simulink model "sampleModel89"  (R2021b)
settings: Solver=VariableStepAuto  StartTime=0.0  StopTime=10.0  RelTol=1e-3
undefined symbols (not defined in the file or in its folder): magnitude
libraries: simulink x7
settings Model: Creator=user  LastModifiedBy=user

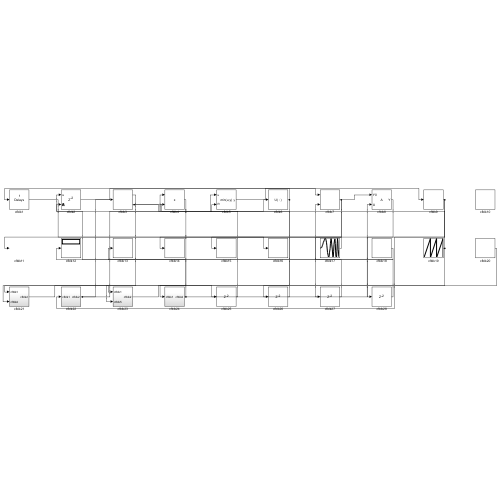
[thumbnail: Simulink's stored preview of the top-level diagram]
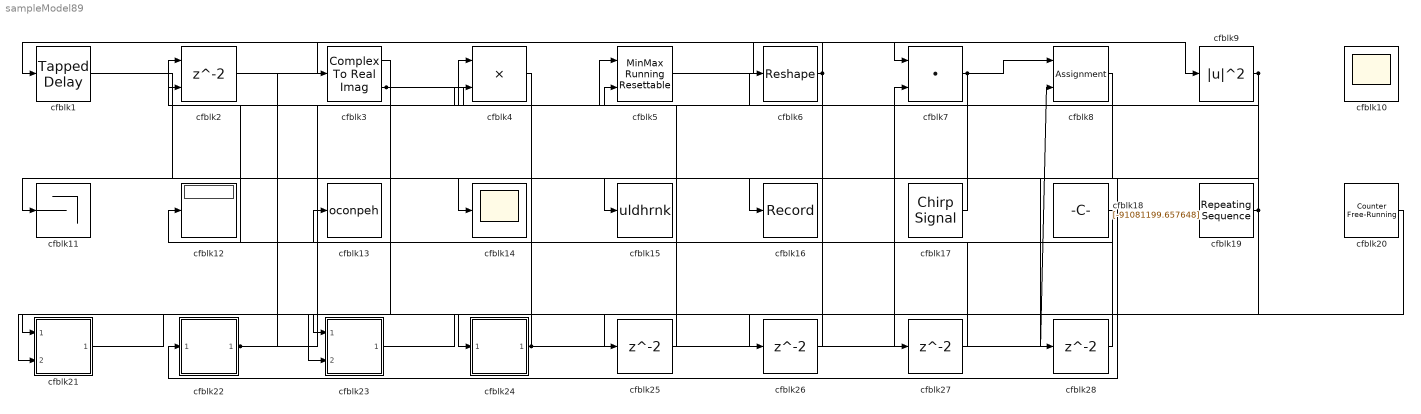
== system sampleModel89 ==
  cfblk1 : simulink/Discrete/Tapped Delay  vinit=0.0  samptime=-1  NumDelays=1  DelayOrder=Oldest  includeCurrent=off
  cfblk10 : Scope
      settings: Floating=on
  cfblk11 : Terminator
  cfblk12 : Display
  cfblk13 : ToWorkspace  VariableName=oconpeh  SaveFormat=Timeseries  SampleTime=-1
  cfblk14 : Scope
  cfblk15 : ToWorkspace  VariableName=uldhrnk  SaveFormat=Timeseries  SampleTime=-1
  cfblk16 : Record  FileSettingsInternal="{\"entries\":[{\"content\":{\"excelSettings\":{\"content\":{},\"type\":\"Streamout.ExcelSettings\"}},\"type\":\"Streamout.FileSettingStorage\",\"uuid\":\"fac87c34-e0b7-4349-b6f4-70da045e78e1\"}],\"packageUris\":[\"http://schema.mathworks.com/mf0/streamout_blocks/R2020a\"],\"version\":\"1.0\"}"  SignalsInternal="{\"entries\":[{\"content\":{\"signals\":[{\"content\":{\"blockPath\":[\"sampleModel89/cfblk16\"],\"channel\":[],\"dimensions\":[1],\"domain\":\"sampleModel89/cfblk16\",\"lineColor\":\"#a2142f\",\"plots\":[1],\"port\":1,\"sid\":[\"\"],\"signalID\":3255,\"signalName\":\"cfblk1\"},\"type\":\"RecordBlkView.Signal\",\"uuid\":\"2643ba45-9ab1-445a-bdcd-ba3203e13d56\"}]},\"type\":\"RecordBlkView.InputSignals\",\"uuid\":\"61955a5d-bbc7-4503-a666-7dac71005f09\"}],\"packageUris\":[\"http://schema.mathworks.com/mf0/streamout_blocks/R2020a\"],\"version\":\"1.0\"}"  VisualizationBindings="{\"sparklinesplugin\":{\"info\":[{\"bindingParametersList\":[],\"subplotID\":1}]}}"
  cfblk17 : simulink/Sources/Chirp Signal  f1=[-255475607.936733]  T=[740321862.264641]  f2=[288984347.187765]
  cfblk18 : Constant  Value=[-91081199.657648]  SampleTime=1
  cfblk19 : simulink/Sources/Repeating Sequence  rep_seq_t=[0 2]  rep_seq_y=[-500814716.924603, 310036400.015080]
  cfblk2 : Delay  ShowEnablePort=on  SampleTime=1
      settings: InputPortMap=u0,e6
  cfblk20 : simulink/Sources/Counter Free-Running  NumBits=[30.000000]  tsamp=-1
  cfblk21 : Subsystem
  cfblk22 : Subsystem
  cfblk23 : Subsystem
  cfblk24 : Subsystem
  cfblk{25..28} (4 alike) : Delay  SampleTime=1
  cfblk3 : ComplexToRealImag
  cfblk4 : Product  Inputs=**
  cfblk5 : simulink/Math Operations/MinMax Running Resettable  Function=min  vinit=0.0
  cfblk6 : Reshape
  cfblk7 : DotProduct  InputSameDT=on  OutDataTypeStr=Inherit: Inherit via internal rule
  cfblk8 : Assignment  DiagnosticForDimensions=Warning  IndexOptions=Index vector (dialog)  Indices=1  OutputSizes=1
  cfblk9 : Math  Operator=magnitude^2  SaturateOnIntegerOverflow=on
  wires:
  cfblk2/1 -> cfblk9/1
  cfblk17/1 -> cfblk11/1
  cfblk18/1 -> cfblk12/1
  cfblk7/1 -> cfblk8/1, cfblk14/1, cfblk26/1
  cfblk5/1 -> cfblk7/1
  cfblk6/1 -> cfblk1/1, cfblk15/1
  cfblk22/1(cfblk2) -> cfblk4/1, cfblk3/1
  cfblk4/1 -> cfblk21/1(cfblk1)
  cfblk24/1(cfblk2) -> cfblk13/1, cfblk8/2
  cfblk9/1 -> cfblk22/1(cfblk1), cfblk28/1
  cfblk1/1 -> cfblk16/1
  cfblk21/1(cfblk2) -> cfblk23/1(cfblk1)
  cfblk19/1 -> cfblk2/1, cfblk24/1(cfblk1)
  cfblk3/1 -> cfblk21/2(cfblk4)
  cfblk3/2 -> cfblk5/2, cfblk6/1
  cfblk20/1 -> cfblk23/2(cfblk5)
  cfblk23/1(cfblk2) -> cfblk25/1
  cfblk25/1 -> cfblk4/2
  cfblk26/1 -> cfblk5/1
  cfblk8/1 -> cfblk27/1
  cfblk27/1 -> cfblk7/2
  cfblk28/1 -> cfblk2/2

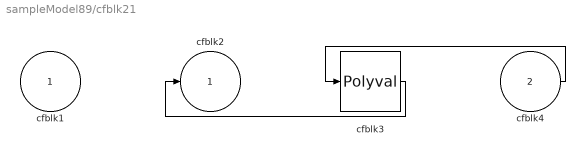
== system sampleModel89/cfblk21 ==
  cfblk1 : Inport
  cfblk4 : Inport  Port=2
  cfblk3 : Polyval  Coefs=[ +2.081618890e-019, -1.441693666e-014, +4.719686976e-010, -8.536869453e-006, +1.621573104e-001, -8.087801117e+001 ]
  cfblk2 : Outport
  wires:
  cfblk4/1 -> cfblk3/1
  cfblk3/1 -> cfblk2/1

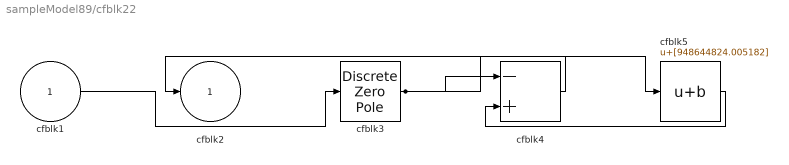
== system sampleModel89/cfblk22 ==
  cfblk1 : Inport
  cfblk3 : DiscreteZeroPole  Poles=[0 0.5]  Gain=1
  cfblk4 : Sum  Inputs=-+
  cfblk5 : Bias  Bias=[948644824.005182]
  cfblk2 : Outport
  wires:
  cfblk4/1 -> cfblk2/1
  cfblk1/1 -> cfblk3/1
  cfblk3/1 -> cfblk4/1, cfblk5/1
  cfblk5/1 -> cfblk4/2

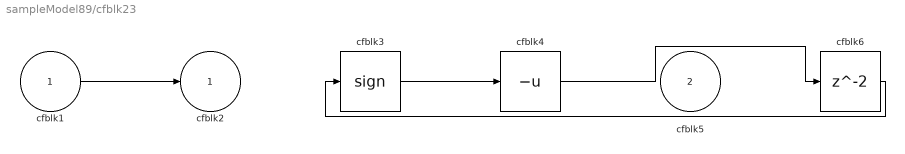
== system sampleModel89/cfblk23 ==
  cfblk1 : Inport
  cfblk5 : Inport  Port=2
  cfblk3 : Signum
  cfblk4 : UnaryMinus
  cfblk6 : Delay  SampleTime=1
  cfblk2 : Outport
  wires:
  cfblk3/1 -> cfblk4/1
  cfblk1/1 -> cfblk2/1
  cfblk4/1 -> cfblk6/1
  cfblk6/1 -> cfblk3/1

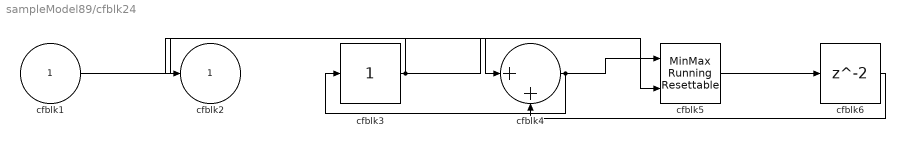
== system sampleModel89/cfblk24 ==
  cfblk1 : Inport
  cfblk3 : simulink/Math Operations/Slider Gain  gain=1  low=0  high=2
  cfblk4 : Sum  Inputs=|++
  cfblk5 : simulink/Math Operations/MinMax Running Resettable  Function=min  vinit=0.0
  cfblk6 : Delay  SampleTime=1
  cfblk2 : Outport
  wires:
  cfblk1/1 -> cfblk4/1
  cfblk4/1 -> cfblk3/1, cfblk5/1
  cfblk3/1 -> cfblk2/1, cfblk5/2
  cfblk5/1 -> cfblk6/1
  cfblk6/1 -> cfblk4/2
